simulink library "Library_Betriebsstrategie"  (R2018b)
settings: Solver=VariableStepAuto  StartTime=0.0  StopTime=10.0  RelTol=1e-3  EnableMultiTasking=on
undefined symbols (not defined in the file): akt_eUELG_HA, akt_eUELG_VA, akt_keinMVS_HA, akt_keinMVS_VA, akt_LSD_HA, akt_LSD_VA, akt_mUELG_HA, akt_mUELG_VA, akt_OD_HA, akt_OD_VA, DiscIntNeverNeededParam, magnitude, mu_road, mu_road_LF, mu_road_LR, mu_road_RF, mu_road_RR, par_MDT, par_VEH, stepsize
libraries: simulink x13
(part 5 of 6)

== system Library_Betriebsstrategie/Momentenverteilung_Lagrange2/Limitierungen gesamt (mit MVS Limits)/Aktuatoren und Delta TV ==
  Aktuator : Constant  Value=par_MDT.AUS.akt.OD_VA
  Aktuator{1..2,6..7} (4 alike) : Constant  Value=0
  Aktuator3 : Constant  Value=par_MDT.AUS.akt.eTV_VA
  Aktuator4 : Constant  Value=par_MDT.AUS.akt.rn_VA
  Aktuator5 : Constant  Value=par_MDT.AUS.akt.OD_HA
  Aktuator8 : Constant  Value=par_MDT.AUS.akt.eTV_HA
  Aktuator9 : Constant  Value=par_MDT.AUS.akt.rn_HA
  Limit elektrisches Überlagerungsgetriebe : Constant  Value=595
  Limit mechanisches Überlagerungsgetriebe1 : Constant  Value=595
  Limit mechanisches Überlagerungsgetriebe2 : Constant  Value=595
  Limit mechanisches Überlagerungsgetriebe3 : Constant  Value=595
  TV Moment pro Achse : MATLAB Function  TreatAsAtomicUnit=on
  Zuweisung Aktuatoren : MATLAB Function  TreatAsAtomicUnit=on
  Delta_T_f : Outport
  Delta_T_r : Outport  Port=2
  A_f : Outport  Port=3
  A_r : Outport  Port=4
  wires:
  Limit mechanisches Überlagerungsgetriebe3/1 -> TV Moment pro Achse/4(L4)
  Limit mechanisches Überlagerungsgetriebe2/1 -> TV Moment pro Achse/3(L3)
  Limit mechanisches Überlagerungsgetriebe1/1 -> TV Moment pro Achse/2(L2)
  Limit elektrisches Überlagerungsgetriebe/1 -> TV Moment pro Achse/1(L1)
  TV Moment pro Achse/2(Delta_T_r) -> Delta_T_r/1
  TV Moment pro Achse/1(Delta_T_f) -> Delta_T_f/1
  Zuweisung Aktuatoren/2(a_r) -> TV Moment pro Achse/7(a_r), A_r/1
  Aktuator/1 -> Zuweisung Aktuatoren/1(A1)
  Aktuator1/1 -> Zuweisung Aktuatoren/2(A2)
  Aktuator2/1 -> Zuweisung Aktuatoren/3(A3)
  Aktuator3/1 -> Zuweisung Aktuatoren/4(A4)
  Aktuator4/1 -> Zuweisung Aktuatoren/5(A5)
  Aktuator5/1 -> Zuweisung Aktuatoren/6(A6)
  Aktuator6/1 -> Zuweisung Aktuatoren/7(A7)
  Aktuator7/1 -> Zuweisung Aktuatoren/8(A8)
  Aktuator8/1 -> Zuweisung Aktuatoren/9(A9)
  Aktuator9/1 -> Zuweisung Aktuatoren/10(A10)
  Zuweisung Aktuatoren/1(a_f) -> TV Moment pro Achse/6(a_f), A_f/1

== system Library_Betriebsstrategie/Momentenverteilung_Regelbasiert/Feedback Controller/Zero Crossing ==
  de0 : Inport
  de1 : Inport  Port=2
  e0 : Inport  Port=3
  e1 : Inport  Port=4
  Product : Product
  Switch : Switch  Criteria=u2 > Threshold
  error(Tc) : Outport
  wires:
  de0/1 -> Product/1
  de1/1 -> Product/2
  Product/1 -> Switch/2
  Switch/1 -> error(Tc)/1
  e1/1 -> Switch/1
  e0/1 -> Switch/3

== system Library_Betriebsstrategie/Momentverteilung_LR/Feedback Controller/Zero Crossing ==
  de0 : Inport
  de1 : Inport  Port=2
  e0 : Inport  Port=3
  e1 : Inport  Port=4
  Product : Product
  Switch : Switch  Criteria=u2 > Threshold
  error(Tc) : Outport
  wires:
  de0/1 -> Product/1
  de1/1 -> Product/2
  Product/1 -> Switch/2
  Switch/1 -> error(Tc)/1
  e1/1 -> Switch/1
  e0/1 -> Switch/3

== system Library_Betriebsstrategie/Momentverteilung_LR/Radmomentenaufteilung/Optimierung links ==
  M_wheel_left : Inport
  Input : Inport  Port=2
  Add2 : Sum  Inputs=-+
  Antriebsleistung R1 : Product  Inputs=**
  Antriebsleistung R2 : Product  Inputs=**
  Bus Selector : BusSelector  OutputSignals=omega.omega_LF,omega.omega_LR
  Constant2 : Constant  Value=60 / (2 * pi)
  Constant3 : Constant  Value=60 / (2 * pi)
  Constant4 : Constant
  Memory : Memory  LinearizeAsDelay=on
  Optimierung links : MATLAB Function  TreatAsAtomicUnit=on
  Product : Product
  Product1 : Product
  Schritte ein Prozent : Constant  Value=0:0.01:1  VectorParams1D=off
  Subsystem : Subsystem
  Triebstrangwirkungsgrad : Lookup_n-D  BreakpointsForDimension1=par_VEH.dt_eta_y  BreakpointsForDimension2=par_VEH.dt_eta_x  Table=par_VEH.dt_eta_z  ExtrapMethod=Clip  UseLastTableValue=on  InternalRulePriority=Speed  RndMeth=Simplest  InputSameDT=on
  Triebstrangwirkungsgrad1 : Lookup_n-D  BreakpointsForDimension1=par_VEH.dt_eta_y  BreakpointsForDimension2=par_VEH.dt_eta_x  Table=par_VEH.dt_eta_z  ExtrapMethod=Clip  UseLastTableValue=on  InternalRulePriority=Speed  RndMeth=Simplest  InputSameDT=on
  Unit Delay : UnitDelay  SampleTime=0.1
  motor_torque : Product  Inputs=*/
  motor_torque1 : Product  Inputs=*/
  transmission_ratio : Constant  Value=par_VEH.dt_i
  transmission_ratio1 : Constant  Value=par_VEH.dt_i
  u_per_min : Product  Inputs=**
  u_per_min1 : Product  Inputs=**
  gamma_left : Outport
  wires:
  Input/1 -> Bus Selector/1
  M_wheel_left/1 -> Product/2, Product1/2, Optimierung links/1(M_wheel_left)
  Bus Selector/1 -> Antriebsleistung R1/1, Optimierung links/2(omega_LF)  "<omega_LF>"
  Bus Selector/2 -> Optimierung links/3(omega_LR), Antriebsleistung R2/1  "<omega_LR>"
  Schritte ein Prozent/1 -> Add2/1, Product/1
  motor_torque/1 -> Triebstrangwirkungsgrad/1
  u_per_min/1 -> Triebstrangwirkungsgrad/2
  Constant3/1 -> Antriebsleistung R1/2
  transmission_ratio/1 -> u_per_min/2, motor_torque/2
  Antriebsleistung R1/1 -> u_per_min/1
  Product/1 -> motor_torque/1
  Triebstrangwirkungsgrad/1 -> Optimierung links/4(eta_LF)  "eta_antr_LF"
  motor_torque1/1 -> Triebstrangwirkungsgrad1/1
  u_per_min1/1 -> Triebstrangwirkungsgrad1/2
  Constant2/1 -> Antriebsleistung R2/2
  transmission_ratio1/1 -> motor_torque1/2, u_per_min1/2
  Antriebsleistung R2/1 -> u_per_min1/1
  Triebstrangwirkungsgrad1/1 -> Optimierung links/5(eta_LR)  "eta_antr_LR"
  Constant4/1 -> Add2/2
  Product1/1 -> motor_torque1/1
  Add2/1 -> Product1/1
  Subsystem/1(gamma_left) -> gamma_left/1, Memory/1
  Memory/1 -> Subsystem/2(gammaL1)
  Optimierung links/2(min_P_loss) -> Unit Delay/1, Subsystem/3(min_Ploss0)
  Optimierung links/1(gammaL) -> Subsystem/1(gammaL0)
  Unit Delay/1 -> Subsystem/4(min_Ploss1)

== system Library_Betriebsstrategie/Momentverteilung_LR/Radmomentenaufteilung/Optimierung rechts ==
  Input : Inport
  M_wheel_right : Inport  Port=2
  Add5 : Sum  Inputs=-+
  Antriebsleistung R3 : Product  Inputs=**
  Antriebsleistung R4 : Product  Inputs=**
  Bus Selector : BusSelector  OutputSignals=omega.omega_RF,omega.omega_RR
  Constant1 : Constant  Value=60 / (2 * pi)
  Constant5 : Constant  Value=60 / (2 * pi)
  Constant6 : Constant
  Memory : Memory  LinearizeAsDelay=on
  Optimierung rechts : MATLAB Function  TreatAsAtomicUnit=on
  Product1 : Product
  Product2 : Product
  Schritte ein Prozent1 : Constant  Value=0:0.01:1  VectorParams1D=off
  Subsystem : Subsystem
  Triebstrangwirkungsgrad2 : Lookup_n-D  BreakpointsForDimension1=par_VEH.dt_eta_y  BreakpointsForDimension2=par_VEH.dt_eta_x  Table=par_VEH.dt_eta_z  ExtrapMethod=Clip  UseLastTableValue=on  InternalRulePriority=Speed  RndMeth=Simplest  InputSameDT=on
  Triebstrangwirkungsgrad3 : Lookup_n-D  BreakpointsForDimension1=par_VEH.dt_eta_y  BreakpointsForDimension2=par_VEH.dt_eta_x  Table=par_VEH.dt_eta_z  ExtrapMethod=Clip  UseLastTableValue=on  InternalRulePriority=Speed  RndMeth=Simplest  InputSameDT=on
  Unit Delay : UnitDelay  SampleTime=0.1
  motor_torque2 : Product  Inputs=*/
  motor_torque3 : Product  Inputs=*/
  transmission_ratio2 : Constant  Value=par_VEH.dt_i
  transmission_ratio3 : Constant  Value=par_VEH.dt_i
  u_per_min2 : Product  Inputs=**
  u_per_min3 : Product  Inputs=**
  gamma_right : Outport
  wires:
  M_wheel_right/1 -> Product2/1, Optimierung rechts/1(M_wheel_right), Product1/1
  Input/1 -> Bus Selector/1
  motor_torque2/1 -> Triebstrangwirkungsgrad2/1
  u_per_min2/1 -> Triebstrangwirkungsgrad2/2
  Constant1/1 -> Antriebsleistung R3/2
  transmission_ratio2/1 -> u_per_min2/2, motor_torque2/2
  Antriebsleistung R3/1 -> u_per_min2/1
  Product1/1 -> motor_torque2/1
  Schritte ein Prozent1/1 -> Add5/1, Product1/2
  Bus Selector/2 -> Antriebsleistung R4/1, Optimierung rechts/3(omega_RR)  "<omega_RR>"
  Bus Selector/1 -> Antriebsleistung R3/1, Optimierung rechts/2(omega_RF)  "<omega_RF>"
  motor_torque3/1 -> Triebstrangwirkungsgrad3/1
  u_per_min3/1 -> Triebstrangwirkungsgrad3/2
  Constant5/1 -> Antriebsleistung R4/2
  transmission_ratio3/1 -> u_per_min3/2, motor_torque3/2
  Antriebsleistung R4/1 -> u_per_min3/1
  Constant6/1 -> Add5/2
  Triebstrangwirkungsgrad3/1 -> Optimierung rechts/4(eta_RR)  "eta_antr_RR"
  Triebstrangwirkungsgrad2/1 -> Optimierung rechts/5(eta_RF)  "eta_antr_RF"
  Product2/1 -> motor_torque3/1
  Add5/1 -> Product2/2
  Subsystem/1(gamma_right) -> gamma_right/1, Memory/1
  Memory/1 -> Subsystem/2(gammaR1)
  Optimierung rechts/2(min_P_loss) -> Unit Delay/1, Subsystem/3(min_Ploss0)
  Optimierung rechts/1(gammaR) -> Subsystem/1(gammaR0)
  Unit Delay/1 -> Subsystem/4(min_Ploss1)

== system Library_Betriebsstrategie/Momentverteilung_LR1/Feedback Controller/Zero Crossing ==
  de0 : Inport
  de1 : Inport  Port=2
  e0 : Inport  Port=3
  e1 : Inport  Port=4
  Product : Product
  Switch : Switch  Criteria=u2 > Threshold
  error(Tc) : Outport
  wires:
  e0/1 -> Switch/3
  e1/1 -> Switch/1
  Switch/1 -> error(Tc)/1
  Product/1 -> Switch/2
  de1/1 -> Product/2
  de0/1 -> Product/1

== system Library_Betriebsstrategie/Momentverteilung_LR1/Radmomentenaufteilung/Optimierung links ==
  M_wheel_left : Inport
  Input : Inport  Port=2
  Add2 : Sum  Inputs=-+
  Antriebsleistung R1 : Product  Inputs=**
  Antriebsleistung R2 : Product  Inputs=**
  Bus Selector : BusSelector  OutputSignals=omega.omega_LF,omega.omega_LR
  Bus Selector1 : BusSelector  OutputSignals=kappa.kappa_LF,vl.vl_LF,kappa.kappa_LR,vl.vl_LR
  Constant2 : Constant  Value=60 / (2 * pi)
  Constant3 : Constant  Value=60 / (2 * pi)
  Constant4 : Constant
  Memory : Memory  LinearizeAsDelay=on
  Optimierung links : MATLAB Function  TreatAsAtomicUnit=on
  Product{,1..3} (4 alike) : Product
  Schritte ein Prozent : Constant  Value=0:0.01:1  VectorParams1D=off
  Subsystem : Subsystem
  Triebstrangwirkungsgrad : Lookup_n-D  BreakpointsForDimension1=par_VEH.dt_eta_y  BreakpointsForDimension2=par_VEH.dt_eta_x  Table=par_VEH.dt_eta_z  ExtrapMethod=Clip  UseLastTableValue=on  InternalRulePriority=Speed  RndMeth=Simplest  InputSameDT=on
  Triebstrangwirkungsgrad1 : Lookup_n-D  BreakpointsForDimension1=par_VEH.dt_eta_y  BreakpointsForDimension2=par_VEH.dt_eta_x  Table=par_VEH.dt_eta_z  ExtrapMethod=Clip  UseLastTableValue=on  InternalRulePriority=Speed  RndMeth=Simplest  InputSameDT=on
  Unit Delay : UnitDelay  SampleTime=0.1
  motor_torque : Product  Inputs=*/
  motor_torque1 : Product  Inputs=*/
  transmission_ratio : Constant  Value=par_VEH.dt_i
  transmission_ratio1 : Constant  Value=par_VEH.dt_i
  u_per_min : Product  Inputs=**
  u_per_min1 : Product  Inputs=**
  gamma_left : Outport
  wires:
  Product3/1 -> Optimierung links/7(v_slip_LR)
  Product2/1 -> Optimierung links/6(v_slip_LF)
  Bus Selector1/4 -> Product3/2  "<vl_LR>"
  Bus Selector1/3 -> Product3/1  "<kappa_LR>"
  Bus Selector1/2 -> Product2/2  "<vl_LF>"
  Bus Selector1/1 -> Product2/1  "<kappa_LF>"
  Unit Delay/1 -> Subsystem/4(min_Ploss1)
  Optimierung links/1(gammaL) -> Subsystem/1(gammaL0)
  Optimierung links/2(min_P_loss) -> Unit Delay/1, Subsystem/3(min_Ploss0)
  Memory/1 -> Subsystem/2(gammaL1)
  Subsystem/1(gamma_left) -> Memory/1, gamma_left/1
  Add2/1 -> Product1/1
  Product1/1 -> motor_torque1/1
  Constant4/1 -> Add2/2
  Triebstrangwirkungsgrad1/1 -> Optimierung links/5(eta_LR)  "eta_antr_LR"
  Antriebsleistung R2/1 -> u_per_min1/1
  transmission_ratio1/1 -> u_per_min1/2, motor_torque1/2
  Constant2/1 -> Antriebsleistung R2/2
  u_per_min1/1 -> Triebstrangwirkungsgrad1/2
  motor_torque1/1 -> Triebstrangwirkungsgrad1/1
  Triebstrangwirkungsgrad/1 -> Optimierung links/4(eta_LF)  "eta_antr_LF"
  Product/1 -> motor_torque/1
  Antriebsleistung R1/1 -> u_per_min/1
  transmission_ratio/1 -> motor_torque/2, u_per_min/2
  Constant3/1 -> Antriebsleistung R1/2
  u_per_min/1 -> Triebstrangwirkungsgrad/2
  motor_torque/1 -> Triebstrangwirkungsgrad/1
  Schritte ein Prozent/1 -> Product/1, Add2/1
  Bus Selector/2 -> Antriebsleistung R2/1, Optimierung links/3(omega_LR)  "<omega_LR>"
  Bus Selector/1 -> Optimierung links/2(omega_LF), Antriebsleistung R1/1  "<omega_LF>"
  M_wheel_left/1 -> Optimierung links/1(M_wheel_left), Product1/2, Product/2
  Input/1 -> Bus Selector/1, Bus Selector1/1

== system Library_Betriebsstrategie/Momentverteilung_LR1/Radmomentenaufteilung/Optimierung rechts ==
  Input : Inport
  M_wheel_right : Inport  Port=2
  Add5 : Sum  Inputs=-+
  Antriebsleistung R3 : Product  Inputs=**
  Antriebsleistung R4 : Product  Inputs=**
  Bus Selector : BusSelector  OutputSignals=omega.omega_RF,omega.omega_RR
  Bus Selector1 : BusSelector  OutputSignals=kappa.kappa_RF,vl.vl_RF,kappa.kappa_RR,vl.vl_RR
  Constant1 : Constant  Value=60 / (2 * pi)
  Constant5 : Constant  Value=60 / (2 * pi)
  Constant6 : Constant
  Memory : Memory  LinearizeAsDelay=on
  Optimierung rechts : MATLAB Function  TreatAsAtomicUnit=on
  Product{1..4} (4 alike) : Product
  Schritte ein Prozent1 : Constant  Value=0:0.01:1  VectorParams1D=off
  Subsystem : Subsystem
  Triebstrangwirkungsgrad2 : Lookup_n-D  BreakpointsForDimension1=par_VEH.dt_eta_y  BreakpointsForDimension2=par_VEH.dt_eta_x  Table=par_VEH.dt_eta_z  ExtrapMethod=Clip  UseLastTableValue=on  InternalRulePriority=Speed  RndMeth=Simplest  InputSameDT=on
  Triebstrangwirkungsgrad3 : Lookup_n-D  BreakpointsForDimension1=par_VEH.dt_eta_y  BreakpointsForDimension2=par_VEH.dt_eta_x  Table=par_VEH.dt_eta_z  ExtrapMethod=Clip  UseLastTableValue=on  InternalRulePriority=Speed  RndMeth=Simplest  InputSameDT=on
  Unit Delay : UnitDelay  SampleTime=0.1
  motor_torque2 : Product  Inputs=*/
  motor_torque3 : Product  Inputs=*/
  transmission_ratio2 : Constant  Value=par_VEH.dt_i
  transmission_ratio3 : Constant  Value=par_VEH.dt_i
  u_per_min2 : Product  Inputs=**
  u_per_min3 : Product  Inputs=**
  gamma_right : Outport
  wires:
  Product4/1 -> Optimierung rechts/2(v_slip_RR)
  Product3/1 -> Optimierung rechts/1(v_slip_RF)
  Bus Selector1/4 -> Product4/2  "<vl_RR>"
  Bus Selector1/3 -> Product4/1  "<kappa_RR>"
  Bus Selector1/2 -> Product3/2  "<vl_RF>"
  Bus Selector1/1 -> Product3/1  "<kappa_RF>"
  Unit Delay/1 -> Subsystem/4(min_Ploss1)
  Optimierung rechts/1(gammaR) -> Subsystem/1(gammaR0)
  Optimierung rechts/2(min_P_loss) -> Unit Delay/1, Subsystem/3(min_Ploss0)
  Memory/1 -> Subsystem/2(gammaR1)
  Subsystem/1(gamma_right) -> Memory/1, gamma_right/1
  Add5/1 -> Product2/2
  Product2/1 -> motor_torque3/1
  Triebstrangwirkungsgrad2/1 -> Optimierung rechts/6(eta_RF)  "eta_antr_RF"
  Triebstrangwirkungsgrad3/1 -> Optimierung rechts/7(eta_RR)  "eta_antr_RR"
  Constant6/1 -> Add5/2
  Antriebsleistung R4/1 -> u_per_min3/1
  transmission_ratio3/1 -> motor_torque3/2, u_per_min3/2
  Constant5/1 -> Antriebsleistung R4/2
  u_per_min3/1 -> Triebstrangwirkungsgrad3/2
  motor_torque3/1 -> Triebstrangwirkungsgrad3/1
  Bus Selector/1 -> Optimierung rechts/4(omega_RF), Antriebsleistung R3/1  "<omega_RF>"
  Bus Selector/2 -> Optimierung rechts/5(omega_RR), Antriebsleistung R4/1  "<omega_RR>"
  Schritte ein Prozent1/1 -> Product1/2, Add5/1
  Product1/1 -> motor_torque2/1
  Antriebsleistung R3/1 -> u_per_min2/1
  transmission_ratio2/1 -> motor_torque2/2, u_per_min2/2
  Constant1/1 -> Antriebsleistung R3/2
  u_per_min2/1 -> Triebstrangwirkungsgrad2/2
  motor_torque2/1 -> Triebstrangwirkungsgrad2/1
  Input/1 -> Bus Selector/1, Bus Selector1/1
  M_wheel_right/1 -> Product1/1, Optimierung rechts/3(M_wheel_right), Product2/1

== system Library_Betriebsstrategie/Momentverteilung_LR2/Feedback Controller/Zero Crossing ==
  de0 : Inport
  de1 : Inport  Port=2
  e0 : Inport  Port=3
  e1 : Inport  Port=4
  Product : Product
  Switch : Switch  Criteria=u2 > Threshold
  error(Tc) : Outport
  wires:
  de0/1 -> Product/1
  de1/1 -> Product/2
  Product/1 -> Switch/2
  Switch/1 -> error(Tc)/1
  e1/1 -> Switch/1
  e0/1 -> Switch/3

== system Library_Betriebsstrategie/Momentverteilung_LR2/Limitierungen gesamt (mit MVS Limits)/Subsystem ==
  a_f : Inport
  a_r : Inport  Port=2
  Limit elektrisches Überlagerungsgetriebe : Constant  Value=595
  Limit mechanisches Überlagerungsgetriebe1 : Constant  Value=595
  Limit mechanisches Überlagerungsgetriebe2 : Constant  Value=595
  Limit mechanisches Überlagerungsgetriebe3 : Constant  Value=595
  MATLAB Function : MATLAB Function  TreatAsAtomicUnit=on
  Delta_T_f : Outport
  Delta_T_r : Outport  Port=2
  wires:
  MATLAB Function/1(Delta_T_f) -> Delta_T_f/1
  MATLAB Function/2(Delta_T_r) -> Delta_T_r/1
  Limit elektrisches Überlagerungsgetriebe/1 -> MATLAB Function/1(L1)
  Limit mechanisches Überlagerungsgetriebe1/1 -> MATLAB Function/2(L2)
  Limit mechanisches Überlagerungsgetriebe2/1 -> MATLAB Function/3(L3)
  Limit mechanisches Überlagerungsgetriebe3/1 -> MATLAB Function/4(L4)
  a_f/1 -> MATLAB Function/6(a_f)
  a_r/1 -> MATLAB Function/7(a_r)

== system Library_Betriebsstrategie/Momentverteilung_LR2/Radmomentenaufteilung/Optimierung links ==
  note: Schlupfgeschwindigkeit
  note: Triebstrangwirkungsgrad
  M_wheel_left : Inport
  Input : Inport  Port=2
  Add2 : Sum  Inputs=-+
  Antriebsleistung R1 : Product  Inputs=**
  Antriebsleistung R2 : Product  Inputs=**
  Bus Selector : BusSelector  OutputSignals=omega.omega_LF,omega.omega_LR
  Bus Selector1 : BusSelector  OutputSignals=kappa.kappa_LF,vl.vl_LF,kappa.kappa_LR,vl.vl_LR
  Bus Selector2 : BusSelector  OutputSignals=Fz.Fz_LF,Fz.Fz_LR,Fs.Fs_LF,Fs.Fs_LR
  Bus to Vector1 : BusToVector
  Bus to Vector18 : BusToVector
  Bus to Vector2 : BusToVector
  Constant2 : Constant  Value=60 / (2 * pi)
  Constant3 : Constant  Value=60 / (2 * pi)
  Constant4 : Constant
  Memory : Memory  LinearizeAsDelay=on
  Optimierung links : MATLAB Function  TreatAsAtomicUnit=on
  Product{,1..3} (4 alike) : Product
  Schritte ein Prozent : Constant  Value=0:0.01:1  VectorParams1D=off
  Subsystem : Subsystem
  To Workspace1 : ToWorkspace  VariableName=sv_vslip_LF  SampleTime=-1
      settings: Decimation=savedec  Save2DSignal=2-D array (concatenate along first dimension)
  To Workspace2 : ToWorkspace  VariableName=sv_vslip_LR  SampleTime=-1
      settings: Decimation=savedec  Save2DSignal=2-D array (concatenate along first dimension)
  To Workspace3 : ToWorkspace  VariableName=sv_Ploss_slipL  SampleTime=-1
      settings: Decimation=savedec  Save2DSignal=2-D array (concatenate along first dimension)
  To Workspace32 : ToWorkspace  VariableName=sv_min_P_lossL  SampleTime=-1
      settings: Decimation=savedec  Save2DSignal=2-D array (concatenate along first dimension)
  To Workspace4 : ToWorkspace  VariableName=sv_Ploss_motL  SampleTime=-1
      settings: Decimation=savedec  Save2DSignal=2-D array (concatenate along first dimension)
  To Workspace5 : ToWorkspace  VariableName=sv_Ploss_tractionL  SampleTime=-1
      settings: Decimation=savedec  Save2DSignal=2-D array (concatenate along first dimension)
  Triebstrangwirkungsgrad : Lookup_n-D  BreakpointsForDimension1=par_VEH.dt_eta_y  BreakpointsForDimension2=par_VEH.dt_eta_x  Table=par_VEH.dt_eta_z  ExtrapMethod=Clip  UseLastTableValue=on  InternalRulePriority=Speed  RndMeth=Simplest  InputSameDT=on
  Triebstrangwirkungsgrad1 : Lookup_n-D  BreakpointsForDimension1=par_VEH.dt_eta_y  BreakpointsForDimension2=par_VEH.dt_eta_x  Table=par_VEH.dt_eta_z  ExtrapMethod=Clip  UseLastTableValue=on  InternalRulePriority=Speed  RndMeth=Simplest  InputSameDT=on
  Unit Delay : UnitDelay  SampleTime=0.1
  motor_torque : Product  Inputs=*/
  motor_torque1 : Product  Inputs=*/
  r_stat0 : Constant  Value=par_VEH.r_stat0
  transmission_ratio : Constant  Value=par_VEH.dt_i
  transmission_ratio1 : Constant  Value=par_VEH.dt_i
  u_per_min : Product  Inputs=**
  u_per_min1 : Product  Inputs=**
  gamma_left : Outport
  wires:
  Optimierung links/3(E) -> To Workspace5/1
  r_stat0/1 -> Optimierung links/12(r)
  Bus Selector2/4 -> Optimierung links/11(Fy_LR)  "<Fs_LR>"
  Bus Selector2/3 -> Optimierung links/10(Fy_LF)  "<Fs_LF>"
  Bus Selector2/2 -> Optimierung links/9(Fz_LR)  "<Fz_LR>"
  Bus Selector2/1 -> Optimierung links/8(Fz_LF)  "<Fz_LF>"
  Input/1 -> Bus Selector2/1, Bus Selector1/1, Bus Selector/1
  M_wheel_left/1 -> Optimierung links/1(M_wheel_left), Product/2, Product1/2
  Bus Selector/1 -> Antriebsleistung R1/1, Optimierung links/2(omega_LF)  "<omega_LF>"
  Bus Selector/2 -> Antriebsleistung R2/1, Optimierung links/3(omega_LR)  "<omega_LR>"
  Schritte ein Prozent/1 -> Add2/1, Product/1
  motor_torque/1 -> Triebstrangwirkungsgrad/1
  u_per_min/1 -> Triebstrangwirkungsgrad/2
  Constant3/1 -> Antriebsleistung R1/2
  transmission_ratio/1 -> u_per_min/2, motor_torque/2
  Antriebsleistung R1/1 -> u_per_min/1
  Product/1 -> motor_torque/1
  Triebstrangwirkungsgrad/1 -> Optimierung links/4(eta_LF)  "eta_antr_LF"
  motor_torque1/1 -> Triebstrangwirkungsgrad1/1
  u_per_min1/1 -> Triebstrangwirkungsgrad1/2
  Constant2/1 -> Antriebsleistung R2/2
  transmission_ratio1/1 -> motor_torque1/2, u_per_min1/2
  Antriebsleistung R2/1 -> u_per_min1/1
  Triebstrangwirkungsgrad1/1 -> Optimierung links/5(eta_LR)  "eta_antr_LR"
  Constant4/1 -> Add2/2
  Product1/1 -> motor_torque1/1
  Add2/1 -> Product1/1
  Subsystem/1(gamma_left) -> gamma_left/1, Memory/1
  Memory/1 -> Subsystem/2(gammaL1)
  Optimierung links/4(gammaL) -> Subsystem/1(gammaL0)
  Unit Delay/1 -> Subsystem/4(min_Ploss1)
  Bus Selector1/1 -> Product2/1  "<kappa_LF>"
  Bus Selector1/2 -> Product2/2  "<vl_LF>"
  Bus Selector1/3 -> Product3/1  "<kappa_LR>"
  Bus Selector1/4 -> Product3/2  "<vl_LR>"
  Bus to Vector18/1 -> To Workspace32/1
  Optimierung links/5(min_P_loss) -> Subsystem/3(min_Ploss0), Unit Delay/1, Bus to Vector18/1
  Bus to Vector1/1 -> To Workspace1/1
  Product2/1 -> Bus to Vector1/1, Optimierung links/6(v_slip_LF)
  Bus to Vector2/1 -> To Workspace2/1
  Product3/1 -> Bus to Vector2/1, Optimierung links/7(v_slip_LR)
  Optimierung links/1(C) -> To Workspace3/1
  Optimierung links/2(D) -> To Workspace4/1

== system Library_Betriebsstrategie/Momentverteilung_LR2/Radmomentenaufteilung/Optimierung rechts ==
  note: Triebstrangwirkungsgrad
  note: Schlupfgeschwindigkeit
  Input : Inport
  M_wheel_right : Inport  Port=2
  Add5 : Sum  Inputs=-+
  Antriebsleistung R3 : Product  Inputs=**
  Antriebsleistung R4 : Product  Inputs=**
  Bus Selector : BusSelector  OutputSignals=omega.omega_RF,omega.omega_RR
  Bus Selector1 : BusSelector  OutputSignals=kappa.kappa_RF,vl.vl_RF,kappa.kappa_RR,vl.vl_RR
  Bus Selector2 : BusSelector  OutputSignals=Fz.Fz_RF,Fz.Fz_RR,Fs.Fs_RF,Fs.Fs_RR
  Bus to Vector1 : BusToVector
  Bus to Vector18 : BusToVector
  Bus to Vector2 : BusToVector
  Constant1 : Constant  Value=60 / (2 * pi)
  Constant5 : Constant  Value=60 / (2 * pi)
  Constant6 : Constant
  Memory : Memory  LinearizeAsDelay=on
  Optimierung rechts : MATLAB Function  TreatAsAtomicUnit=on
  Product{1..4} (4 alike) : Product
  Schritte ein Prozent1 : Constant  Value=0:0.01:1  VectorParams1D=off
  Subsystem : Subsystem
  To Workspace1 : ToWorkspace  VariableName=sv_vslip_RF  SampleTime=-1
      settings: Decimation=savedec  Save2DSignal=2-D array (concatenate along first dimension)
  To Workspace2 : ToWorkspace  VariableName=sv_vslip_RR  SampleTime=-1
      settings: Decimation=savedec  Save2DSignal=2-D array (concatenate along first dimension)
  To Workspace3 : ToWorkspace  VariableName=sv_Ploss_slipR  SampleTime=-1
      settings: Decimation=savedec  Save2DSignal=2-D array (concatenate along first dimension)
  To Workspace32 : ToWorkspace  VariableName=sv_min_P_lossR  SampleTime=-1
      settings: Decimation=savedec  Save2DSignal=2-D array (concatenate along first dimension)
  To Workspace4 : ToWorkspace  VariableName=sv_Ploss_motR  SampleTime=-1
      settings: Decimation=savedec  Save2DSignal=2-D array (concatenate along first dimension)
  To Workspace5 : ToWorkspace  VariableName=sv_Ploss_tractionR  SampleTime=-1
      settings: Decimation=savedec  Save2DSignal=2-D array (concatenate along first dimension)
  Triebstrangwirkungsgrad2 : Lookup_n-D  BreakpointsForDimension1=par_VEH.dt_eta_y  BreakpointsForDimension2=par_VEH.dt_eta_x  Table=par_VEH.dt_eta_z  ExtrapMethod=Clip  UseLastTableValue=on  InternalRulePriority=Speed  RndMeth=Simplest  InputSameDT=on
  Triebstrangwirkungsgrad3 : Lookup_n-D  BreakpointsForDimension1=par_VEH.dt_eta_y  BreakpointsForDimension2=par_VEH.dt_eta_x  Table=par_VEH.dt_eta_z  ExtrapMethod=Clip  UseLastTableValue=on  InternalRulePriority=Speed  RndMeth=Simplest  InputSameDT=on
  Unit Delay : UnitDelay  SampleTime=0.1
  motor_torque2 : Product  Inputs=*/
  motor_torque3 : Product  Inputs=*/
  r_stat0 : Constant  Value=par_VEH.r_stat0
  transmission_ratio2 : Constant  Value=par_VEH.dt_i
  transmission_ratio3 : Constant  Value=par_VEH.dt_i
  u_per_min2 : Product  Inputs=**
  u_per_min3 : Product  Inputs=**
  gamma_right : Outport
  wires:
  r_stat0/1 -> Optimierung rechts/12(r)
  Bus Selector2/4 -> Optimierung rechts/11(Fy_RR)  "<Fs_RR>"
  Bus Selector2/3 -> Optimierung rechts/10(Fy_RF)  "<Fs_RF>"
  Bus Selector2/2 -> Optimierung rechts/9(Fz_RR)  "<Fz_RR>"
  Bus Selector2/1 -> Optimierung rechts/8(Fz_RF)  "<Fz_RF>"
  Optimierung rechts/3(E) -> To Workspace5/1
  M_wheel_right/1 -> Product2/1, Optimierung rechts/1(M_wheel_right), Product1/1
  Input/1 -> Bus Selector1/1, Bus Selector/1, Bus Selector2/1
  motor_torque2/1 -> Triebstrangwirkungsgrad2/1
  u_per_min2/1 -> Triebstrangwirkungsgrad2/2
  Constant1/1 -> Antriebsleistung R3/2
  transmission_ratio2/1 -> u_per_min2/2, motor_torque2/2
  Antriebsleistung R3/1 -> u_per_min2/1
  Product1/1 -> motor_torque2/1
  Schritte ein Prozent1/1 -> Add5/1, Product1/2
  Bus Selector/2 -> Optimierung rechts/3(omega_RR), Antriebsleistung R4/1  "<omega_RR>"
  Bus Selector/1 -> Optimierung rechts/2(omega_RF), Antriebsleistung R3/1  "<omega_RF>"
  motor_torque3/1 -> Triebstrangwirkungsgrad3/1
  u_per_min3/1 -> Triebstrangwirkungsgrad3/2
  Constant5/1 -> Antriebsleistung R4/2
  transmission_ratio3/1 -> u_per_min3/2, motor_torque3/2
  Antriebsleistung R4/1 -> u_per_min3/1
  Constant6/1 -> Add5/2
  Triebstrangwirkungsgrad3/1 -> Optimierung rechts/5(eta_RR)  "eta_antr_RR"
  Triebstrangwirkungsgrad2/1 -> Optimierung rechts/4(eta_RF)  "eta_antr_RF"
  Product2/1 -> motor_torque3/1
  Add5/1 -> Product2/2
  Subsystem/1(gamma_right) -> gamma_right/1, Memory/1
  Memory/1 -> Subsystem/2(gammaR1)
  Optimierung rechts/4(gammaR) -> Subsystem/1(gammaR0)
  Unit Delay/1 -> Subsystem/4(min_Ploss1)
  Bus Selector1/1 -> Product3/1  "<kappa_RF>"
  Bus Selector1/2 -> Product3/2  "<vl_RF>"
  Bus Selector1/3 -> Product4/1  "<kappa_RR>"
  Bus Selector1/4 -> Product4/2  "<vl_RR>"
  Bus to Vector18/1 -> To Workspace32/1
  Optimierung rechts/5(min_P_loss) -> Subsystem/3(min_Ploss0), Unit Delay/1, Bus to Vector18/1
  Bus to Vector1/1 -> To Workspace1/1
  Product3/1 -> Optimierung rechts/6(v_slip_RF), Bus to Vector1/1
  Bus to Vector2/1 -> To Workspace2/1
  Product4/1 -> Optimierung rechts/7(v_slip_RR), Bus to Vector2/1
  Optimierung rechts/1(C) -> To Workspace3/1
  Optimierung rechts/2(D) -> To Workspace4/1

== system Library_Betriebsstrategie/Momentverteilung_LR/Radmomentenaufteilung/Optimierung links/Subsystem ==
  gammaL0 : Inport
  gammaL1 : Inport  Port=2
  min_Ploss0 : Inport  Port=3
  min_Ploss1 : Inport  Port=4
  Add : Sum  Inputs=+-
  Gain : Gain  Gain=1.001
  Switch : Switch
  gamma_left : Outport
  wires:
  Switch/1 -> gamma_left/1
  min_Ploss1/1 -> Add/2
  Gain/1 -> Add/1
  min_Ploss0/1 -> Gain/1
  Add/1 -> Switch/2
  gammaL0/1 -> Switch/3
  gammaL1/1 -> Switch/1

== system Library_Betriebsstrategie/Momentverteilung_LR/Radmomentenaufteilung/Optimierung rechts/Subsystem ==
  gammaR0 : Inport
  gammaR1 : Inport  Port=2
  min_Ploss0 : Inport  Port=3
  min_Ploss1 : Inport  Port=4
  Add : Sum  Inputs=+-
  Gain : Gain  Gain=1.001
  Switch : Switch
  gamma_right : Outport
  wires:
  Switch/1 -> gamma_right/1
  min_Ploss1/1 -> Add/2
  Gain/1 -> Add/1
  min_Ploss0/1 -> Gain/1
  Add/1 -> Switch/2
  gammaR0/1 -> Switch/3
  gammaR1/1 -> Switch/1

== system Library_Betriebsstrategie/Momentverteilung_LR1/Radmomentenaufteilung/Optimierung links/Subsystem ==
  gammaL0 : Inport
  gammaL1 : Inport  Port=2
  min_Ploss0 : Inport  Port=3
  min_Ploss1 : Inport  Port=4
  Add : Sum  Inputs=+-
  Gain : Gain  Gain=1.001
  Switch : Switch
  gamma_left : Outport
  wires:
  gammaL1/1 -> Switch/1
  gammaL0/1 -> Switch/3
  Add/1 -> Switch/2
  min_Ploss0/1 -> Gain/1
  Gain/1 -> Add/1
  min_Ploss1/1 -> Add/2
  Switch/1 -> gamma_left/1

== system Library_Betriebsstrategie/Momentverteilung_LR1/Radmomentenaufteilung/Optimierung rechts/Subsystem ==
  gammaR0 : Inport
  gammaR1 : Inport  Port=2
  min_Ploss0 : Inport  Port=3
  min_Ploss1 : Inport  Port=4
  Add : Sum  Inputs=+-
  Gain : Gain  Gain=1.001
  Switch : Switch
  gamma_right : Outport
  wires:
  gammaR1/1 -> Switch/1
  gammaR0/1 -> Switch/3
  Add/1 -> Switch/2
  min_Ploss0/1 -> Gain/1
  Gain/1 -> Add/1
  min_Ploss1/1 -> Add/2
  Switch/1 -> gamma_right/1

== system Library_Betriebsstrategie/Momentverteilung_LR2/Radmomentenaufteilung/Optimierung links/Subsystem ==
  gammaL0 : Inport
  gammaL1 : Inport  Port=2
  min_Ploss0 : Inport  Port=3
  min_Ploss1 : Inport  Port=4
  Add : Sum  Inputs=+-
  Gain : Gain  Gain=1.005
  Switch : Switch
  gamma_left : Outport
  wires:
  Switch/1 -> gamma_left/1
  min_Ploss1/1 -> Add/2
  Gain/1 -> Add/1
  min_Ploss0/1 -> Gain/1
  Add/1 -> Switch/2
  gammaL0/1 -> Switch/3
  gammaL1/1 -> Switch/1

== system Library_Betriebsstrategie/Momentverteilung_LR2/Radmomentenaufteilung/Optimierung rechts/Subsystem ==
  gammaR0 : Inport
  gammaR1 : Inport  Port=2
  min_Ploss0 : Inport  Port=3
  min_Ploss1 : Inport  Port=4
  Add : Sum  Inputs=+-
  Gain : Gain  Gain=1.005
  Switch : Switch
  gamma_right : Outport
  wires:
  Switch/1 -> gamma_right/1
  min_Ploss1/1 -> Add/2
  Gain/1 -> Add/1
  min_Ploss0/1 -> Gain/1
  Add/1 -> Switch/2
  gammaR0/1 -> Switch/3
  gammaR1/1 -> Switch/1

== matlab function Library_Betriebsstrategie/Momentverteilung_LR1/Radmomentenaufteilung/Optimierung links/Optimierung links ==
  data: M_wheel_left input; omega_LF input; omega_LR input; gammaL output; eta_LF input; eta_LR input; min_P_loss output; v_slip_LF input; v_slip_LR input
function [gammaL, min_P_loss] = fcn(M_wheel_left, omega_LF, omega_LR, eta_LF, eta_LR, v_slip_LF, v_slip_LR)

%% Diskrete Variable x (1 Prozent Schritte für Radmomentverteilung)
step = 0.01;
x = [0:step:1];
n = 1/step + 1;
Einser = ones(1,n);

%% Leistungsverluste in Abhängigkeit vom Antreiben oder Rekuperieren
if M_wheel_left >= 0 %vorne
    P_loss_f = ((Einser ./ eta_LF - 1)*omega_LF*M_wheel_left) .* x;
else
    P_loss_f = ((1 - eta_LF)*omega_LF*M_wheel_left) .* x;
end

if M_wheel_left >= 0 %hinten
    P_loss_r = ((Einser ./ eta_LR - 1)*omega_LR*M_wheel_left) .* (1-x);
else
    P_loss_r = ((1 - eta_LR)*omega_LR*M_wheel_left) .* (1-x);
end

%% Leistungsverluste in Abhängigkeit des Radschlupfes (also wird Traktion auch mit berücksichtigt)
P_slip_f = abs(v_slip_LF * M_wheel_left) .* x;

P_slip_r = abs(v_slip_LR * M_wheel_left) .* (1-x);

%% Minimum der diskreten Leistungsverluste
P_loss = P_loss_f + P_loss_r + P_slip_f + P_slip_r;
[A, B] = min(P_loss);

%% Wertezuweisung
gammaL = step*B - step;
min_P_loss = A;

== matlab function Library_Betriebsstrategie/Momentenverteilung_Regelbasiert/Radmomentenaufteilung/Optimale Verteilung ==
  data: FxlimFR input; FxFR output; FxlimFL input; FxFL output; FxRR output; FxRL output; FxlimRR input; FxlimRL input; DeltaTV input; DriverReq input; FzFR input; FzFL input; FzRR input; FzRL input
function [FxFR,FxFL,FxRR,FxRL] = RegelbasierteAufteilung(FxlimFR,FxlimFL,FxlimRR,FxlimRL,DeltaTV,DriverReq,FzFR,FzFL,FzRR,FzRL)
    %Longitudinal (Priority)
    F_f=DriverReq*((FzFR+FzFL)/(FzRR+FzRL+FzFR+FzFL));
    F_r=DriverReq*(1-((FzFR+FzFL)/(FzRR+FzRL+FzFR+FzFL)));
    FxFR=F_f*0.5;
    FxFL=F_f*0.5;
    FxRR=F_r*0.5;
    FxRL=F_r*0.5;
    flag=0;
    if abs(FxFL)>FxlimFL || abs(FxFR)>FxlimFR
        FxFL=min(FxlimFL,FxlimFR)*sign(DriverReq);
        FxFR=FxFL;
        dF_rear=F_f-FxFR-FxFL;
        dF_RR=dF_rear*0.5;
        dF_RL=dF_rear*0.5;
        FxRR=FxRR+dF_RR;
        FxRL=FxRL+dF_RL;
        flag=1;
    end
    if abs(FxRL)>FxlimRL || abs(FxRR)>FxlimRR
        FxRL=min(FxlimRL,FxlimRR)*sign(DriverReq);
        FxRR=FxRL;
        flag=1;
    end
    %Lateral Control
    if DeltaTV>0 && flag==1
        TVf=DeltaTV*(FzFR/(FzFR+FzRR));
        TVr=DeltaTV*(FzRR/(FzRR+FzFR));
        FxFR=FxFR+TVf;
        FxRR=FxRR+TVr;
        if abs(FxFR)>FxlimFR
            dTV=abs(FxFR)-FxlimFR;
            FxFR=FxlimFR;
        end
        if abs(FxRR)>FxlimRR
            FxRR=FxlimRR;
        end
    end
    if DeltaTV<0 && flag==1
        TVf=abs(DeltaTV*(FzFL/(FzFL+FzRL)));
        TVr=abs(DeltaTV*(FzRL/(FzFL+FzRL)));
        FxFL=FxFL+TVf;
        FxRL=FxRL+TVf;
        if abs(FxFL)>FxlimFL
            dTV=abs(FxFL)-FxlimFL;
            FxFL=FxlimFL;
        end
        if abs(FxRL)>FxlimRL
            FxRL=FxlimRL;
        end
    end
    if DeltaTV>0 && flag==0
        dF_split=DeltaTV/2;
        if dF_split>min((FxlimFR-FxFR+FxlimRR-FxRR),(FxlimFL+FxFL+FxlimRL+FxRL))
            dF_split=min((FxlimFR-FxFR+FxlimRR-FxRR),(FxlimFL+FxFL+FxlimRL+FxRL));
        end
        FxFR=FxFR+dF_split*(FzFR/(FzRR+FzFR));
        FxRR=FxRR+dF_split*(FzRR/(FzRR+FzFR));
        if FxFR>FxlimFR
            dFr=FxFR-FxlimFR;
            FxFR=FxlimFR;
            FxRR=FxRR+dFr;
            if FxRR>FxlimRR
                FxRR=FxlimRR;
            end
        end
        FxFL=FxFL-dF_split*(FzFL/(FzFL+FzRL));
        FxRL=FxRL-dF_split*(FzRL/(FzRL+FzFL));
        if abs(FxFL)>FxlimFL
            dFl=abs(FxFL)-FxlimFL;
            FxFL=-FxlimFL;
            FxRL=-FxRL-dFl;
            if abs(FxRL)>FxlimRL
                FxRL=-FxlimRL;
            end
        end
    end
    if DeltaTV<0 && flag==0
     dF_split=DeltaTV/2;
        if dF_split>min((FxlimFL-FxFL+FxlimRL-FxRL),(FxlimFR+FxFR+FxlimRR+FxRR))
            dF_split=min((FxlimFL-FxFL+FxlimRL-FxRL),(FxlimFR+FxFR+FxlimRR+FxRR));
        end
        FxFL=FxFL+dF_split*(FzFL/(FzRL+FzFL));
        FxRR=FxRL+dF_split*(FzRL/(FzRL+FzFL));
        if FxFL>FxlimFL
            dFl=FxFL-FxlimFL;
            FxFL=FxlimFL;
            FxRL=FxRL+dFl;
            if FxRL>FxlimRL
                FxRL=FxlimRL;
            end
        end
        FxFR=FxFR-dF_split*(FzFR/(FzFR+FzRR));
        FxRR=FxRR-dF_split*(FzRR/(FzRR+FzFR));
        if abs(FxFR)>FxlimFR
            dFr=abs(FxFR)-FxlimFR;
            FxFR=-FxlimFR;
            FxRR=-FxRR-dFr;
            if abs(FxRR)>FxlimRR
                FxRR=-FxlimRR;
            end
        end
    end

== matlab function Library_Betriebsstrategie/Momentverteilung_LR/Radmomentenaufteilung/Optimierung links/Optimierung links ==
  data: M_wheel_left input; omega_LF input; omega_LR input; gammaL output; eta_LF input; eta_LR input; min_P_loss output
function [gammaL, min_P_loss] = fcn(M_wheel_left, omega_LF, omega_LR, eta_LF, eta_LR)

%% Diskrete Variable x (1 Prozent Schritte für Radmomentverteilung)
step = 0.01;
x = [0:step:1];
n = 1/step + 1;
Einser = ones(1,n);

%% Leistungsverluste in Abhängigkeit vom Antreiben oder Rekuperieren
if M_wheel_left >= 0 %vorne
    P_loss_f = ((Einser ./ eta_LF - 1)*omega_LF*M_wheel_left) .* x;
else
    P_loss_f = ((1 - eta_LF)*omega_LF*M_wheel_left) .* x;
end

if M_wheel_left >= 0 %hinten
    P_loss_r = ((Einser ./ eta_LR - 1)*omega_LR*M_wheel_left) .* (1-x);
else
    P_loss_r = ((1 - eta_LR)*omega_LR*M_wheel_left) .* (1-x);
end


%% Minimum der diskreten Leistungsverluste
P_loss = P_loss_f + P_loss_r;
[A, B] = min(P_loss);

%% Wertezuweisung
gammaL = step*B - step;
min_P_loss = A;

== matlab function Library_Betriebsstrategie/Momentverteilung_LR1/Radmomentenaufteilung/Optimierung rechts/Optimierung rechts ==
  data: v_slip_RF input; v_slip_RR input; M_wheel_right input; omega_RF input; omega_RR input; eta_RF input; eta_RR input; gammaR output; min_P_loss output
function [gammaR, min_P_loss] = fcn(v_slip_RF, v_slip_RR, M_wheel_right, omega_RF, omega_RR, eta_RF, eta_RR)

%% Diskrete Variable x (1 Prozent Schritte für Radmomentverteilung)
step = 0.01;
x = [0:step:1];
n = 1/step + 1;
Einser = ones(1,n);

%% Leistungsverluste in Abhängigkeit vom Antreiben oder Rekuperieren
if M_wheel_right >= 0 %vorne
    P_loss_f = ((Einser ./ eta_RF - 1)*omega_RF*M_wheel_right) .* x;
else
    P_loss_f = ((1 - eta_RF)*omega_RF*M_wheel_right) .* x;
end

if M_wheel_right >= 0 %hinten
    P_loss_r = ((Einser ./ eta_RR - 1)*omega_RR*M_wheel_right) .* (1-x);
else
    P_loss_r = ((1 - eta_RR)*omega_RR*M_wheel_right) .* (1-x);
end

%% Leistungsverluste in Abhängigkeit des Radschlupfes (also wird Traktion auch mit berücksichtigt)
P_slip_f = abs(v_slip_RF * M_wheel_right) .* x;

P_slip_r = abs(v_slip_RR * M_wheel_right) .* (1-x);

%% Minimum der diskreten Leistungsverluste
P_loss = P_loss_f + P_loss_r + P_slip_f + P_slip_r;
[A, B] = min(P_loss);

%% Wertezuweisung
gammaR = step*B - step;
min_P_loss = A;

== matlab function Library_Betriebsstrategie/Momentverteilung_LR/Radmomentenaufteilung/Optimierung rechts/Optimierung rechts ==
  data: M_wheel_right input; omega_RF input; omega_RR input; eta_RR input; gammaR output; eta_RF input; min_P_loss output
function [gammaR, min_P_loss] = fcn(M_wheel_right, omega_RF, omega_RR, eta_RR, eta_RF)

%% Diskrete Variable x (1 Prozent Schritte für Radmomentverteilung)
step = 0.01;
x = [0:step:1];
n = 1/step + 1;
Einser = ones(1,n);

%% Leistungsverluste in Abhängigkeit vom Antreiben oder Rekuperieren
if M_wheel_right >= 0 %vorne
    P_loss_f = ((Einser ./ eta_RF - 1)*omega_RF*M_wheel_right) .* x;
else
    P_loss_f = ((1 - eta_RF)*omega_RF*M_wheel_right) .* x;
end

if M_wheel_right >= 0 %hinten
    P_loss_r = ((Einser ./ eta_RR - 1)*omega_RR*M_wheel_right) .* (1-x);
else
    P_loss_r = ((1 - eta_RR)*omega_RR*M_wheel_right) .* (1-x);
end

%% Minimum der diskreten Leistungsverluste
P_loss = P_loss_f + P_loss_r;
[A, B] = min(P_loss);

%% Wertezuweisung
gammaR = step*B - step;
min_P_loss = A;

== matlab function Library_Betriebsstrategie/Momentenverteilung_Diskret/Radmomentenaufteilung/Diskrete Optimierung ==
  data: A1 output; A2 output; A3 output; A4 output; A5 output; M_wheel input; Mz input; r input; s05 input; omega_LF input; omega_LR input; omega_RF input; omega_RR input; M_RF output; eta_LF input; eta_LR input; M_LF output; M_RR output; M_LR output; eta_RF input; eta_RR input; Fz_LF input; Fz_LR input; Fz_RF input; Fz_RR input; Fy_LF input; Fy_LR input; Fy_RF input; Fy_RR input; vslip_LF input; vslip_LR input; vslip_RF input; vslip_RR input; Falt_LF input; Falt_LR input; Falt_RF input; Falt_RR input
function [A1, A2, A3, A4, A5, M_RF, M_LF, M_RR, M_LR] = fcn(M_wheel, Mz, r, s05, omega_LF, omega_LR, omega_RF, omega_RR, eta_LF, eta_LR, eta_RF, eta_RR, Fz_LF, Fz_LR, Fz_RF, Fz_RR, Fy_LF, Fy_LR, Fy_RF, Fy_RR, vslip_LF, vslip_LR, vslip_RF, vslip_RR, Falt_LF, Falt_LR, Falt_RF, Falt_RR)

%% Diskrete Variable x (1 Prozent Schritte für Radmomentverteilung)
step = 0.01;
x = [0:step:1];
xt = transpose(x);
n = 1/step + 1;
Einser = ones(n,n);

%% Kräfte am Rad
Fx = M_wheel/r;
F_TV = Mz/s05;

Fx_LF = xt*x*Fx;        % Achtung die Kräfte werden hier  durch eine gesamte Matrix dargestellt
Fx_RF = xt*(1-x)*Fx;    % In der Ausgabe sind die Kräfte skalare Werte und heißen F_LF usw.
Fx_LR = (1-xt)*x*Fx;
Fx_RR = (1-xt)*(1-x)*Fx; % Erzeugen einer nxn Matrix über Vektormultiplikation nx1 * 1xn

%% Leistungsverluste in Abhängigkeit vom Antreiben oder Rekuperieren
if M_wheel >= 0 %vorne links
    P_loss_LF = ((Einser ./ eta_LF - 1)*omega_LF) .* Fx_LF *r;
else
    P_loss_LF = ((1 - eta_LF)*omega_LF) .* Fx_LF *r;
end

if M_wheel >= 0 %vorne rechts
    P_loss_RF = ((Einser ./ eta_RF - 1)*omega_RF) .* Fx_RF *r;
else
    P_loss_RF = ((1 - eta_RF)*omega_RF) .* Fx_RF *r;
end

if M_wheel >= 0 %hinten links
    P_loss_LR = ((Einser ./ eta_LR - 1)*omega_LR) .* Fx_LR *r;
else
    P_loss_LR = ((1 - eta_LR)*omega_LR) .* Fx_LR *r;
end

if M_wheel >= 0 %hinten rechts
    P_loss_RR = ((Einser ./ eta_RR - 1)*omega_RR) .* Fx_RR *r;
else
    P_loss_RR = ((1 - eta_RR)*omega_RR) .* Fx_RR *r;
end

%% Leistungsverluste über die Schlupfgeschwindigkeit
P_slip_LF = abs(vslip_LF) .* abs(Fx_LF);
P_slip_LR = abs(vslip_LR) .* abs(Fx_LR);
P_slip_RF = abs(vslip_RF) .* abs(Fx_RF);
P_slip_RR = abs(vslip_RR) .* abs(Fx_RR);

%% Minimale Ausnutzung des Traktionspotentials
mueT_LF = ((Fx_LF.^2 + Fy_LF^2) ./ Fz_LF).^0.5;
mueT_LR = ((Fx_LR.^2 + Fy_LR^2) ./ Fz_LR).^0.5;
mueT_RF = ((Fx_RF.^2 + Fy_RF^2) ./ Fz_RF).^0.5;
mueT_RR = ((Fx_RR.^2 + Fy_RR^2) ./ Fz_RR).^0.5;

%% Stabilität der Lösung bzw. Verhindern von übermäßigem Springen
P_delta = 0.01*(abs(Fx_LF-Falt_LF)+abs(Fx_LR-Falt_LR)+abs(Fx_RF-Falt_RF)+abs(Fx_RR-Falt_RR));

%% Berücksichtigung des TV Moments
P_TV = 0.001*((Fx_LF*(-s05)+Fx_RF*s05+Fx_LR*(-s05)+Fx_RR*s05)-Mz).^2;

%% !!! Minimum der diskreten Leistungsverluste bzw. der gesamten Zielfunktion !!!

P_min = P_TV + 1*(P_slip_LF + P_slip_LR + P_slip_RF + P_slip_RR)+ 1*(mueT_LF+mueT_LR+mueT_RF+mueT_RR) + P_delta;

%% Wertezuweisung
[minval,idx]=min(P_min(:));
[aidx,bidx]=ind2sub(size(P_min),idx);

gamma = step*aidx - step;
gammaF = step*bidx - step;

F_LF = gamma*gammaF*Fx;
F_RF = gamma*(1-gammaF)*Fx;
F_LR = (1-gamma)*gammaF*Fx;
F_RR = (1-gamma)*(1-gammaF)*Fx;

M_LF = F_LF*r;
M_RF = F_RF*r;
M_LR = F_LR*r;
M_RR = F_RR*r;

%% Analyse der einzelnen Anteile des Leistungsverlustes
%A1 = ((F_LF*(-s05)+F_RF*s05+F_LR*(-s05)+F_RR*s05)-Mz)^2;
%A2 = (abs(F_LF-Falt_LF)+abs(F_LR-Falt_LR)+abs(F_RF-Falt_RF)+abs(F_RR-Falt_RR));
%A3 = abs(vslip_LF).*abs(F_LF) + abs(vslip_LR).*abs(F_LR) + abs(vslip_RF).*abs(F_RF) + abs(vslip_RR).*abs(F_RR);
%A4 = ((F_LF.^2 + Fy_LF^2) ./ Fz_LF).^0.5 + ((F_LR.^2 + Fy_LR^2) ./ Fz_LR).^0.5 + ((F_RF.^2 + Fy_RF^2) ./ Fz_RF).^0.5 + ((F_RR.^2 + Fy_RR^2) ./ Fz_RR).^0.5;

A1=P_TV;
A2=P_delta;
A3=(P_slip_LF + P_slip_LR + P_slip_RF + P_slip_RR);
A4=1*(mueT_LF+mueT_LR+mueT_RF+mueT_RR);
A5=P_min;

== matlab function Library_Betriebsstrategie/Momentenverteilung_Lagrange/Radmomentenaufteilung/Optimierung mit Lagrange Multiplikator Methode ==
  data: tF input; tR input; lf input; lr input; delta input; X_req input; Mz input; X_FL output; X_FR output; X_RL output; X_RR output; Z_FL input; Z_FR input; Z_RL input; Z_RR input; X_FL1 input; X_FR1 input; X_RL1 input; X_RR1 input
function [X_FL, X_FR, X_RL, X_RR] = fcn(tF, tR, lf, lr, delta, X_req, Mz, Z_FL, Z_FR, Z_RL, Z_RR, X_FL1, X_FR1, X_RL1, X_RR1)


%% Matrix für die Randbedingungen ( Gesamtmoment und TV Moment)
B0 = [cos(delta) cos(delta) 1 1; (-tF/2)*cos(delta)+lf*sin(delta) (tF/2)*cos(delta)+lf*sin(delta) -tR/2 tR/2];
y0 = [X_req; Mz];

%% Algorythmus
    %% Initialbedingungen
i=0;    
B=B0;
y=y0;
     
    %% Verhindern abgehobener Räder
if Z_FL < 1
    Z_FL = 1;
    x_FL_max = 0;
end

if Z_FR < 1
    Z_FR = 1;
    x_FR_max = 0;
end

if Z_RL < 1
    Z_RL = 1;
    x_RL_max = 0;
end

if Z_RR < 1
    Z_RR = 1;
    x_RR_max = 0;
end

%% Matrizen für die Mimimierung
W1 = [1/Z_FL 0 0 0; 0 1/Z_FR 0 0; 0 0 1/Z_RL 0; 0 0 0 1/Z_RR];
W2 = 0.01 * eye(4);
W = W1 + W2;
X_alt = [X_FL1; X_FR1; X_RL1; X_RR1];

%% Berechnung von Xij
G = (W^(-2))*(B')*(B*(W^(-2))*(B'))^(-1);
X = G*y + (eye(4)-G*B)*(W^(-2))*(W2^2)*X_alt;

%% Limits berücksichtigen
    
    
    
%% Ausgabewerte berechnen
X_FL = X(1);
X_FR = X(2);
X_RL = X(3);
X_RR = X(4);

== matlab function Library_Betriebsstrategie/Momentverteilung_LR2/Limitierungen gesamt (mit MVS Limits)/Limits Zusammenführung ==
  data: FxlimRF input; FxlimLF input; FxlimRR input; Fx_LF_ub output; Fx_LF_lb output; Fx_RF_ub output; Fx_RF_lb output; Fx_LR_ub output; Fx_LR_lb output; Fx_RR_ub output; Fx_RR_lb output; FxlimLR input; M_RF_ub input; M_RF_lb input; M_LF_ub input; M_LF_lb input; M_RR_ub input; M_RR_lb input; M_LR_ub input; M_LR_lb input; M_F_lb input; M_F_ub input; M_R_lb input; M_R_ub input; DELTA_T_f input; DELTA_T_r input; a_f input; a_r input; r input
function [Fx_LF_ub, Fx_LF_lb, Fx_RF_ub, Fx_RF_lb, Fx_LR_ub, Fx_LR_lb, Fx_RR_ub, Fx_RR_lb] = fcn(FxlimRF, FxlimLF, FxlimRR, FxlimLR, M_RF_ub, M_RF_lb, M_LF_ub, M_LF_lb, M_RR_ub, M_RR_lb, M_LR_ub, M_LR_lb, M_F_lb, M_F_ub, M_R_lb, M_R_ub,DELTA_T_f, DELTA_T_r,a_f, a_r, r)


Fx_LF_ub = FxlimLF;
Fx_RF_ub = FxlimRF;
Fx_LF_lb = (-1*FxlimLF);
Fx_RF_lb = (-1*FxlimRF);

Fx_LR_ub = FxlimLR;
Fx_RR_ub = FxlimRR;
Fx_LR_lb = (-1*FxlimLR);
Fx_RR_lb = (-1*FxlimRR);
    
%% Nomenklatur der Aktuatoren a_r und a_f
    % 1 = nur Elektromaschinen an der Achse
    % 2 = Offenes Differential an der Achse
    % 3 = Limited Slip Differential an der Achse
    % 4 = Elektrisches Überlagerungsgetriebe an der Achse
    % 5 = Mechanisches Überlagerungsgetriebe an der Achse
 
    
%% Nur Elektromotoren: Limit ist Minimum/Maximum aus Reifenlimit und Limit der EM
if a_f == 1
    Fx_LF_ub = min(FxlimLF,(M_LF_ub/r));
    Fx_RF_ub = min(FxlimRF,(M_RF_ub/r));
    Fx_LF_lb = max((-1*FxlimLF),(M_LF_lb/r));
    Fx_RF_lb = max((-1*FxlimRF),(M_RF_lb/r));
end

if a_r == 1
    Fx_LR_ub = min(FxlimLR,(M_LR_ub/r));
    Fx_RR_ub = min(FxlimRR,(M_RR_ub/r));
    Fx_LR_lb = max((-1*FxlimLR),(M_LR_lb/r));
    Fx_RR_lb = max((-1*FxlimRR),(M_RR_lb/r));
end

%% Offenes Differential: Limit ist Minimum/Maximum aus Reifenlimit und genau der Hälfte des max. Moments der achszentralen EM
if a_f == 2
    Fx_LF_ub = min(FxlimLF,(0.5*M_F_ub/r));
    Fx_RF_ub = min(FxlimRF,(0.5*M_F_ub/r));
    Fx_LF_lb = max((-1*FxlimLF),(0.5*M_F_lb/r));
    Fx_RF_lb = max((-1*FxlimRF),(0.5*M_F_lb/r));
end

if a_r == 2
    Fx_LR_ub = min(FxlimLR,(0.5*M_R_ub/r));
    Fx_RR_ub = min(FxlimRR,(0.5*M_R_ub/r));
    Fx_LR_lb = max((-1*FxlimLR),(0.5*M_R_lb/r));
    Fx_RR_lb = max((-1*FxlimRR),(0.5*M_R_lb/r));
end

%% Limited Slip Differential:
if a_f >= 3 
    Fx_LF_ub = min(FxlimLF,(0.5*M_F_ub/r + 0.5*DELTA_T_f/r));
    Fx_RF_ub = min(FxlimRF,(0.5*M_F_ub/r + 0.5*DELTA_T_f/r));
    Fx_LF_lb = max((-1*FxlimLF),(0.5*M_F_lb/r - 0.5*DELTA_T_f/r));
    Fx_RF_lb = max((-1*FxlimRF),(0.5*M_F_lb/r - 0.5*DELTA_T_f/r));
end

if a_r >= 3
    Fx_LR_ub = min(FxlimLR,(0.5*M_R_ub/r + 0.5*DELTA_T_r/r));
    Fx_RR_ub = min(FxlimRR,(0.5*M_R_ub/r + 0.5*DELTA_T_r/r));
    Fx_LR_lb = max((-1*FxlimLR),(0.5*M_R_lb/r - 0.5*DELTA_T_r/r));
    Fx_RR_lb = max((-1*FxlimRR),(0.5*M_R_lb/r - 0.5*DELTA_T_r/r));
end


%% Elektrisches Überlagerungsgetriebe


%% Mechanisches Überlagerungsgetriebe

== matlab function Library_Betriebsstrategie/Momentverteilung_LR2/Radmomentenaufteilung/Optimierung links/Optimierung links ==
  data: C output; D output; E output; M_wheel_left input; omega_LF input; omega_LR input; gammaL output; eta_LF input; eta_LR input; min_P_loss output; v_slip_LF input; v_slip_LR input; Fz_LF input; Fz_LR input; Fy_LF input; Fy_LR input; r input
function [C, D, E, gammaL, min_P_loss] = fcn(M_wheel_left, omega_LF, omega_LR, eta_LF, eta_LR, v_slip_LF, v_slip_LR, Fz_LF, Fz_LR, Fy_LF, Fy_LR, r)

%% Diskrete Variable x (1 Prozent Schritte für Radmomentverteilung) und Initialisierung
step = 0.01;
x = [0:step:1];
n = 1/step + 1;
Einser = ones(1,n);
K_loss = 1;
K_slip = 1;
K_traction = 10;

%% Leistungsverluste in Abhängigkeit vom Antreiben oder Rekuperieren
if M_wheel_left >= 0 %vorne
    P_loss_f = ((Einser ./ eta_LF - 1)*omega_LF*M_wheel_left) .* x;
else
    P_loss_f = ((1 - eta_LF)*omega_LF*M_wheel_left) .* x;
end

if M_wheel_left >= 0 %hinten
    P_loss_r = ((Einser ./ eta_LR - 1)*omega_LR*M_wheel_left) .* (1-x);
else
    P_loss_r = ((1 - eta_LR)*omega_LR*M_wheel_left) .* (1-x);
end

%% Leistungsverluste in Abhängigkeit des Radschlupfes (also wird Traktion auch mit berücksichtigt)
P_slip_f = 5* abs(v_slip_LF * M_wheel_left/r) .* x;

P_slip_r = 5* abs(v_slip_LR * M_wheel_left/r) .* (1-x);

%% Ausnutzung des Kraftführungspotentials
mueT_LF = ((((M_wheel_left/r).*x).^2 + Fy_LF^2) ./ Fz_LF).^0.5;
mueT_LR = ((((M_wheel_left/r).*(1-x)).^2 + Fy_LR^2) ./ Fz_LR).^0.5;

%% Minimum der diskreten Leistungsverluste
P_loss = K_loss*(P_loss_f + P_loss_r) + K_slip*(P_slip_f + P_slip_r) + K_traction*(mueT_LF + mueT_LR);
[A, B] = min(P_loss);

%% Wertezuweisung
gammaL = step*B - step;
min_P_loss = A;

%% Analyse der Gewichtung bzw der Anteile an der Minimierungsfunktion
P_slip_links = K_slip*(P_slip_f + P_slip_r);
P_loss_links = K_loss*(P_loss_f + P_loss_r);
P_traction_links = K_traction*(mueT_LF + mueT_LR);
[C] = min(P_slip_links);
[D] = min(P_loss_links);
[E] = min(P_traction_links);

== matlab function Library_Betriebsstrategie/Schaltstrategie/Radmoment zu Motormoment ==
  data: i_LF input; i_RF input; i_LR input; i_RR input; i_F input; i_R input; M_LF input; m_LF output; M_RF input; M_LR input; M_RR input; m_RF output; m_LR output; m_RR output; m_F output; m_R output
function [m_LF, m_RF, m_LR, m_RR, m_F, m_R] = fcn(i_LF, i_RF, i_LR, i_RR, i_F, i_R, M_LF, M_RF, M_LR, M_RR)

%% Motormoment Achszentraler Aufbau
m_F=(M_LF+M_RF)/i_F;
m_R=(M_LR+M_RR)/i_R;

%% Motormoment Radindividueller Aufbau
m_LF=M_LF/i_LF;
m_RF=M_RF/i_RF;
m_LR=M_LR/i_LR;
m_RR=M_RR/i_RR;
